simulink library "MyLibrary"  (R2022a)
settings: Solver=VariableStepAuto  StartTime=0.0  StopTime=10.0  RelTol=1e-3
values from neighbouring files (symbols this model uses):
  Vf = 0.6    [LLC_Resonant_Converter_v1_data.m]    (also in OBC_v1_data.m; Totem_Pole_PFC_v1_data.m)
undefined symbols (not defined in the file or in its folder): Cs_fet, gcbh, Rs_fet, sps_rtmsupport
libraries: spsDiodeModel x1, spsIdealSwitchModel x1
settings Model: Creator=Client  LastModifiedBy=brune
settings DebuggingCC: SaveWithParameterizedLinksMsg=none
settings ModelReferenceCC: EnableRefExpFcnMdlSchedulingChecks=off
settings RTWCC: Description=Generic Real-Time Target

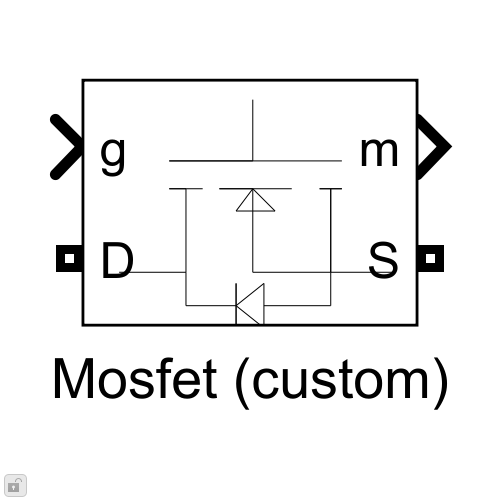
[thumbnail: Simulink's stored preview of the top-level diagram]
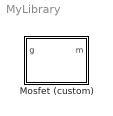
== system MyLibrary ==
  Mosfet (custom) : Subsystem  DialogController=POWERSYS.PowerSysDialog  LoadFcn=sps_rtmsupport('LoadFcn',gcbh);  StartFcn=sps_rtmsupport('StartFcn',gcbh);  StopFcn=sps_rtmsupport('StopFcn',gcbh);  mask(Custom FET){Ron=1e-3, Lon=0, Rd=1e-3, Vfd=Vf, IC=0, Rs=Rs_fet, Cs=Cs_fet, Measurements=on}
      mask prompts: Ron "FET resistance Ron (Ohms) :"; Lon "Internal diode inductance Lon (H) :"; Rd "Internal diode resistance Rd  (Ohms) :"; Vfd "Internal diode forward voltage Vf (V) :"; IC "Initial current Ic (A) :"; Rs "Snubber resistance Rs (Ohms) :"; Cs "Snubber capacitance Cs (F) :"; Measurements "Show measurement port"
      mask help: FET and internal diode in parallel with a series RC snubber circuit. When a gate signal is applied the MOSFET conducts and acts as a resistance (Ron) in both directions. If the gate signal falls to zero when current is negative, current is transferred to the antiparallel diode.
      mask init:
      | block = gcb;
      | [WantBlockChoice,Ts,X,Y,Ron] = powericon('SwitchesInit','MOSFET',block,Rs,Cs,Ron);
      | Csnubber  = Cs;
      settings: CopyFcn=sps_rtmsupport('CopyFcn',gcbh);  DeleteFcn=sps_rtmsupport('DeleteFcn',gcbh);  UndoDeleteFcn=sps_rtmsupport('UndoDeleteFcn',gcbh);  ModelCloseFcn=sps_rtmsupport('ModelCloseFcn',gcbh);  PreSaveFcn=sps_rtmsupport('PreSaveFcn',gcbh);  PostSaveFcn=sps_rtmsupport('PostSaveFcn',gcbh);  NameChangeFcn=sps_rtmsupport('NameChangeFcn',gcbh);  PreCopyFcn=sps_rtmsupport('PreCopyFcn',gcbh);  OpenFcn=sps_rtmsupport('OpenFcn',gcbh, 8);  CloseFcn=sps_rtmsupport('CloseFcn',gcbh);  PreDeleteFcn=sps_rtmsupport('PreDeleteFcn',gcbh);
      mask Help: helpview(psbhelp);
      mask Callback Ron: powericon('SwitchesEnables',gcb,'MOSFET');
      mask Display: plot(X.p1,Y.p1,X.p2,Y.p2,X.p3,Y.p3,X.p4,Y.p4,X.p5,Y.p5,X.p6,Y.p6,X.p7,Y.p7,X.p8,Y.p8)

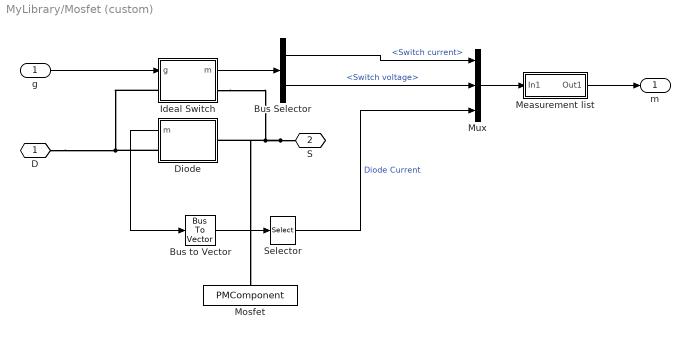
== system MyLibrary/Mosfet (custom) ==
  g : Inport
  Bus Selector : BusSelector  OutputSignals=Switch current,Switch voltage
  Bus to Vector : BusToVector
  Diode : Subsystem  DialogController=POWERSYS.PowerSysDialog  LoadFcn=sps_rtmsupport('LoadFcn',gcbh);  StartFcn=sps_rtmsupport('StartFcn',gcbh);  StopFcn=sps_rtmsupport('StopFcn',gcbh);  mask(Diode){Ron=Rd, Lon=Lon, Vf=Vfd, IC=0, UseSnubber=off, Rs=inf, Cs=0, Measurements=on}
      mask prompts: Ron "Resistance Ron (Ohms) :"; Lon "Inductance Lon (H) :"; Vf "Forward voltage Vf (V) :"; IC "Initial current Ic (A) :"; UseSnubber "Snubber"; Rs "Snubber resistance Rs (Ohms) :"; Cs "Snubber capacitance Cs (F) :"; Measurements "Show measurement port"
      mask help:
      | Implements a diode in parallel with a series RC snubber circuit.
      | In on-state the Diode model has an internal resistance (Ron) and inductance (Lon).
      | For most applications the internal inductance should be set to zero.
      | The Diode impedance is infinite in off-state mode.
      mask init:
      | block = gcb;
      | [WantBlockChoice,Ts,X,Y,Ron,Vf] = powericon('SwitchesInit','Diode',block,Rs,Cs,Ron,Vf);
      | powericon('SetInternalModels','set',block,WantBlockChoice);
      settings: CopyFcn=sps_rtmsupport('CopyFcn',gcbh); powericon('SwitchesCopyFcn','Diode',gcb)  DeleteFcn=sps_rtmsupport('DeleteFcn',gcbh);  UndoDeleteFcn=sps_rtmsupport('UndoDeleteFcn',gcbh);  ModelCloseFcn=sps_rtmsupport('ModelCloseFcn',gcbh);  PreSaveFcn=sps_rtmsupport('PreSaveFcn',gcbh);  PostSaveFcn=sps_rtmsupport('PostSaveFcn',gcbh);  NameChangeFcn=sps_rtmsupport('NameChangeFcn',gcbh);  PreCopyFcn=sps_rtmsupport('PreCopyFcn',gcbh);  OpenFcn=sps_rtmsupport('OpenFcn',gcbh, [5 8]);  CloseFcn=sps_rtmsupport('CloseFcn',gcbh);  PreDeleteFcn=sps_rtmsupport('PreDeleteFcn',gcbh);
      mask Help: helpview(psbhelp);
      mask Callback Ron: powericon('SwitchesEnables',gcb,'Diode');
      mask Callback Measurements:
      | powericon('OutputMCback',gcb);
      | %sps_rtmsupport('parametereditingmodes',gcbh, [5 8]);
      mask Display: plot(X.p1,Y.p1,X.p2,Y.p2,X.p3,Y.p3,X.p4,Y.p4,X.p5,Y.p5,X.p6,Y.p6)
  Ideal Switch : Subsystem  DialogController=POWERSYS.PowerSysDialog  LoadFcn=sps_rtmsupport('LoadFcn',gcbh);  StartFcn=sps_rtmsupport('StartFcn',gcbh);  StopFcn=sps_rtmsupport('StopFcn',gcbh);  mask(Ideal Switch){Ron=Ron, Lon=0, IC=0, Rs=Rs, Cs=Csnubber, Measurements=on}
      mask prompts: Ron "Internal resistance Ron (Ohms) :"; Lon "Inductance Lon (H) :"; IC "Initial state (0 for 'open', 1 for 'closed') :"; Rs "Snubber resistance Rs (Ohms) :"; Cs "Snubber capacitance Cs (F) :"; Measurements "Show measurement port"
      mask help:
      | Switch controlled by a gate signal in parallel with a series RC snubber circuit.
      | In on-state the Switch model has an internal resistance (Ron).
      |  In off-state this internal resistance is infinite.
      | The internal resistance must be greater than zero.
      | The switch model is on-state when the gate signal (g) is set to 1.
      mask init:
      | block = gcb;
      | [WantBlockChoice,Ts,X,Y,Ron] = powericon('SwitchesInit','Ideal Switch',block,Rs,Cs,Ron);
      | powericon('SetInternalModels','set',block,WantBlockChoice);
      settings: CopyFcn=sps_rtmsupport('CopyFcn',gcbh); powericon('SwitchesCopyFcn','Ideal Switch',gcb)  DeleteFcn=sps_rtmsupport('DeleteFcn',gcbh);  UndoDeleteFcn=sps_rtmsupport('UndoDeleteFcn',gcbh);  ModelCloseFcn=sps_rtmsupport('ModelCloseFcn',gcbh);  PreSaveFcn=sps_rtmsupport('PreSaveFcn',gcbh);  PostSaveFcn=sps_rtmsupport('PostSaveFcn',gcbh);  NameChangeFcn=sps_rtmsupport('NameChangeFcn',gcbh);  PreCopyFcn=sps_rtmsupport('PreCopyFcn',gcbh);  OpenFcn=sps_rtmsupport('OpenFcn',gcbh, 6);  CloseFcn=sps_rtmsupport('CloseFcn',gcbh);  PreDeleteFcn=sps_rtmsupport('PreDeleteFcn',gcbh);
      mask Help: helpview(psbhelp);
      mask Callback Ron: powericon('SwitchesEnables',gcb,'Ideal Switch');
      mask Callback Measurements: powericon('OutputMCback',gcb);
      mask Display: plot(X.p1,Y.p1,X.p2,Y.p2,X.p3,Y.p3,X.p4,Y.p4,X.p5,Y.p5)
  Measurement list : Subsystem
  Mosfet : PMComponent  PhysicalDomain=powersysdomain  LeftPortType=p1  RightPortType=p1  LConnTagsString=a  RConnTagsString=__new0  mask(InnerPowersysBlock){}
      mask Display: disp('SPS internal use\nDo not delete')
  Mux : Mux  Inputs=3
  Selector : Selector  InputPortWidth=2  IndexOptions=Index vector (dialog)  Indices=1  OutputSizes=1
  D : PMIOPort  Side=Left
  S : PMIOPort  Port=2  Side=Right
  m : Outport  VectorParamsAs1DForOutWhenUnconnected=off
  wires:
  Mux/1 -> Measurement list/1(In1)
  Selector/1 -> Mux/3  "Diode Current"
  Diode/1(m) -> Bus to Vector/1
  Ideal Switch/1(m) -> Bus Selector/1
  g/1 -> Ideal Switch/1(g)
  Measurement list/1(Out1) -> m/1
  Bus to Vector/1 -> Selector/1
  Bus Selector/2 -> Mux/2  "<Switch voltage>"
  Bus Selector/1 -> Mux/1  "<Switch current>"
  connections:
  Diode/RConn1 -- D/RConn1 -- Ideal Switch/LConn1
  S/RConn1 -- Diode/LConn1 -- Mosfet/LConn1 -- Ideal Switch/RConn1

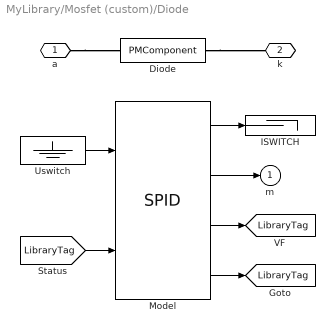
== system MyLibrary/Mosfet (custom)/Diode ==
  Diode : PMComponent  PhysicalDomain=powersysdomain  LeftPortType=p1  RightPortType=p1  LConnTagsString=a  RConnTagsString=__new0  mask(InnerPowersysBlock){}
      mask Display: disp('SPS internal use\nDo not delete')
  ISWITCH : Terminator
  Model : spsDiodeModel/SPID  SystemSampleTime=-1  VariantActivationTime=update diagram  Latency=0  AutoFrameSizeCalculation=off
  Uswitch : Ground
  a : PMIOPort  Side=Left
  k : PMIOPort  Port=2  Side=Right
  m : Outport  VectorParamsAs1DForOutWhenUnconnected=off
  tag scope: LibraryTag=global
  wires:
  Model/2 -> m/1
  [LibraryTag] -> Model/2
  Model/3 -> [LibraryTag]
  Model/4 -> [LibraryTag]
  Model/1 -> ISWITCH/1
  Uswitch/1 -> Model/1
  connections:
  Diode/RConn1 -- k/RConn1
  a/RConn1 -- Diode/LConn1

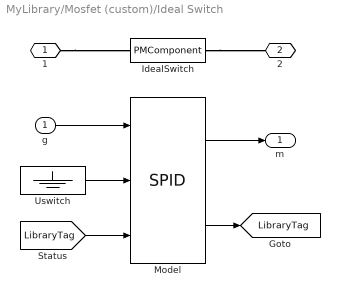
== system MyLibrary/Mosfet (custom)/Ideal Switch ==
  g : Inport
  IdealSwitch : PMComponent  PhysicalDomain=powersysdomain  LeftPortType=p1  RightPortType=p1  LConnTagsString=a  RConnTagsString=__new0  mask(InnerPowersysBlock){}
      mask Display: disp('SPS internal use\nDo not delete')
  Model : spsIdealSwitchModel/SPID  SystemSampleTime=-1  VariantActivationTime=update diagram  Latency=0  AutoFrameSizeCalculation=off
  Uswitch : Ground
  1 : PMIOPort  Side=Left
  2 : PMIOPort  Port=2  Side=Right
  m : Outport  VectorParamsAs1DForOutWhenUnconnected=off
  tag scope: LibraryTag=global
  wires:
  g/1 -> Model/1
  Model/1 -> m/1
  [LibraryTag] -> Model/3
  Model/2 -> [LibraryTag]
  Uswitch/1 -> Model/2
  connections:
  IdealSwitch/RConn1 -- 2/RConn1
  1/RConn1 -- IdealSwitch/LConn1

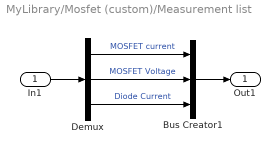
== system MyLibrary/Mosfet (custom)/Measurement list ==
  In1 : Inport
  Bus Creator1 : BusCreator  Inputs=3
  Demux : Demux  Outputs=[1,1,1]
  Out1 : Outport  VectorParamsAs1DForOutWhenUnconnected=off
  wires:
  In1/1 -> Demux/1
  Bus Creator1/1 -> Out1/1
  Demux/1 -> Bus Creator1/1  "MOSFET current"
  Demux/2 -> Bus Creator1/2  "MOSFET Voltage"
  Demux/3 -> Bus Creator1/3  "Diode Current"
